simulink model "Sliding Mode Control"  (R2021a)
settings: Solver=VariableStepAuto  StartTime=0.0  StopTime=30
libraries: simulink x3
settings Model: SimulationMode=accelerator  Creator=victo  LastModifiedBy=victo

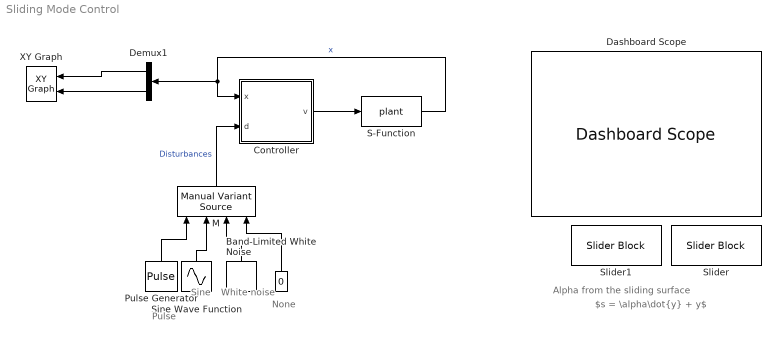
== system Sliding Mode Control ==
  note: $s = \alpha\dot{y} + y$
  note: Alpha from the sliding surface
  note: White noise
  note: Pulse
  note: Sine
  note: None
  " " : Constant  Value=0
  Band-Limited White Noise : simulink/Sources/Band-Limited White Noise  Cov=[0.1]  Ts=0.0002  seed=[23341]
  Controller : Subsystem
  Dashboard Scope : DashboardScope
  Demux1 : Demux  Outputs=2
  M : simulink/Signal Routing/Manual Variant Source  NumChoices=4  LabelModeActiveChoice=V_4
  Pulse Generator : DiscretePulseGenerator  PulseType=Time based  Amplitude=11  Period=1000
  S-Function : S-Function  FunctionName=plant  SFunctionDeploymentMode=off  EnableBusSupport=off
  Sine Wave Function : Sin  Amplitude=11  SampleTime=0
  Slider : SliderBlock
  Slider1 : SliderBlock  ScaleMax=10
  XY Graph : simulink/Sinks/XY Graph  xmin=-15  xmax=15  ymin=-15  ymax=15  st=-1
  wires:
  Controller/1(v) -> S-Function/1
  Pulse Generator/1 -> M/1
  " "/1 -> M/4
  Band-Limited White Noise/1 -> M/3
  Sine Wave Function/1 -> M/2
  M/1 -> Controller/2(d)  "Disturbances"
  Demux1/1 -> XY Graph/1
  Demux1/2 -> XY Graph/2
  S-Function/1 -> Demux1/1, Controller/1(x)  "x"

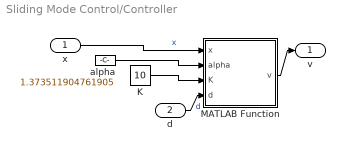
== system Sliding Mode Control/Controller ==
  x : Inport
  d : Inport  Port=2
  K : Constant  Value=10
  MATLAB Function : MATLAB Function  TreatAsAtomicUnit=on
  alpha : Constant  Value=1.373511904761905
  v : Outport
  wires:
  MATLAB Function/1(v) -> v/1
  alpha/1 -> MATLAB Function/2(alpha)
  K/1 -> MATLAB Function/3(K)
  d/1 -> MATLAB Function/4(d)  "d"
  x/1 -> MATLAB Function/1(x)  "x"

== matlab function Sliding Mode Control/Controller/MATLAB Function ==
  data: x input; v output; alpha input; K input; d input
function v = SMC(x, alpha, K, d)
x1 = x(1);
x2 = x(2);    
f_hat = x1 + x2 - 2*x1^3;
s = x1 + alpha*x2; %Sliding surface 

sfun = sign(s); %Classical option

%For a smoother control you could use
% sfun = tanh(s)

%or, for example,

% epsilon = 0.001; %%With epsilon going to 0, sfunc (below) would be = to sign(s)
%sfun = s/(abs(s) + epsilon) %%Saturaded  

v = -(x2/alpha - f_hat + K*sfun/alpha) + d;
